simulink model "bldc_mod_1"  (R2019b)
settings: Solver=VariableStepAuto  StartTime=0.0  StopTime=10.0  RelTol=1e-3
InitFcn:
  | R =1.2;
  | L =0.056;
  | J = 0.00095;
  | b =0.002;
settings Model: Creator=srikesh  LastModifiedBy=srikesh

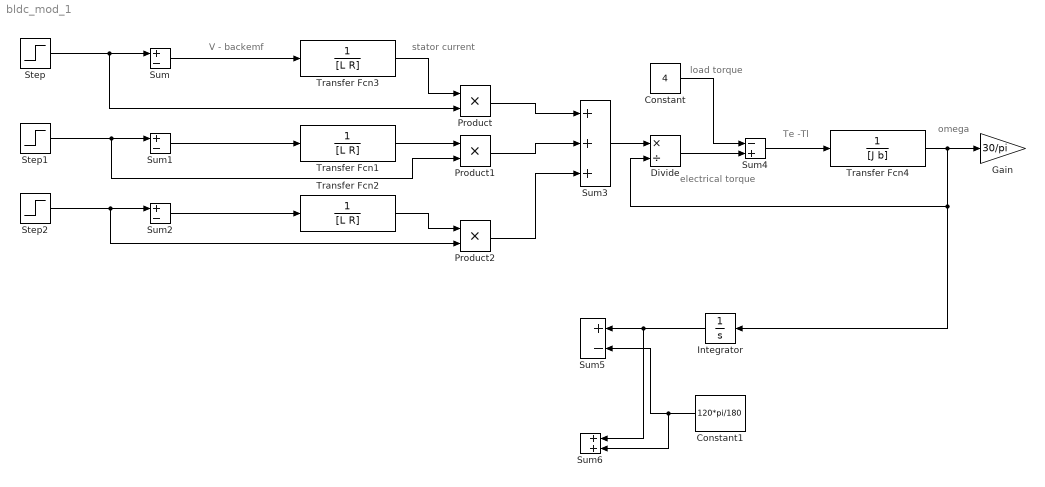
== system bldc_mod_1 ==
  note: omega
  note: stator current
  note: V - backemf
  note: Te -Tl
  note: electrical torque
  note: load torque
  Constant : Constant  Value=4
  Constant1 : Constant  Value=120*pi/180
  Divide : Product  Inputs=*/
  Gain : Gain  Gain=30/pi
  Integrator : Integrator
  Product : Product
  Product1 : Product
  Product2 : Product
  Step : Step  SampleTime=0
  Step1 : Step  SampleTime=0
  Step2 : Step  SampleTime=0
  Sum{,1..2,5} (4 alike) : Sum  Inputs=+-
  Sum3 : Sum  Inputs=+++
  Sum4 : Sum  Inputs=-+
  Sum6 : Sum
  Transfer Fcn1 : TransferFcn  Denominator=[L R]
  Transfer Fcn2 : TransferFcn  Denominator=[L R]
  Transfer Fcn3 : TransferFcn  Denominator=[L R]
  Transfer Fcn4 : TransferFcn  Denominator=[J b]
  wires:
  Step/1 -> Product/2, Sum/1
  Step1/1 -> Product1/2, Sum1/1
  Step2/1 -> Product2/2, Sum2/1
  Sum/1 -> Transfer Fcn3/1
  Sum1/1 -> Transfer Fcn1/1
  Sum2/1 -> Transfer Fcn2/1
  Transfer Fcn3/1 -> Product/1
  Transfer Fcn1/1 -> Product1/1
  Transfer Fcn2/1 -> Product2/1
  Product/1 -> Sum3/1
  Product1/1 -> Sum3/2
  Product2/1 -> Sum3/3
  Sum3/1 -> Divide/1
  Divide/1 -> Sum4/2
  Constant/1 -> Sum4/1
  Sum4/1 -> Transfer Fcn4/1
  Transfer Fcn4/1 -> Divide/2, Integrator/1, Gain/1
  Integrator/1 -> Sum6/1, Sum5/1
  Constant1/1 -> Sum6/2, Sum5/2
